simulink model "yaw_damper"  (R2022b)
settings: Solver=VariableStepAuto  StartTime=0.0  StopTime=100  RelTol=1e-3
values from neighbouring files (symbols this model uses):
  G_b_drda = [G_a*G_bdr*(1-k_dr*G_s*G_f*G_rdr_hat), G_a*G_bda-k_dr*G_f*G_s*G_a*G_bdr*G_rda_hat]    [dynamic_SAS_lat.m]
  G_b_drdano = [G_a*G_bdr*(1-k_dr*G_s*G_f*G_rdr_hatno), G_a*G_bda-k_dr*G_f*G_s*G_a*G_bdr*G_rda_hatno]    [dynamic_SAS_lat.m]
  G_phi_drda = [G_a*G_phidr*(1-k_dr*G_s*G_f*G_rdr_hat), G_a*G_phida-k_dr*G_s*G_f*G_a*G_phidr*G_rda_hat]    [dynamic_SAS_lat.m]
  G_phi_drdano = [G_a*G_phidr*(1-k_dr*G_s*G_f*G_rdr_hatno), G_a*G_phida-k_dr*G_s*G_f*G_a*G_phidr*G_rda_hatno]    [dynamic_SAS_lat.m]
libraries: cstblocks x6, simulink_extras x4
settings Model: Creator=mluser  LastModifiedBy=mluser

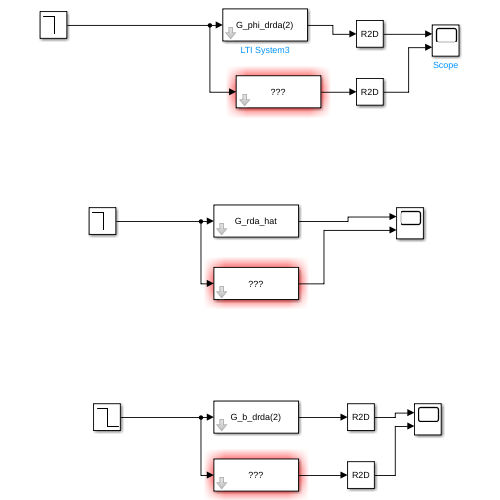
[thumbnail: Simulink's stored preview of the top-level diagram]
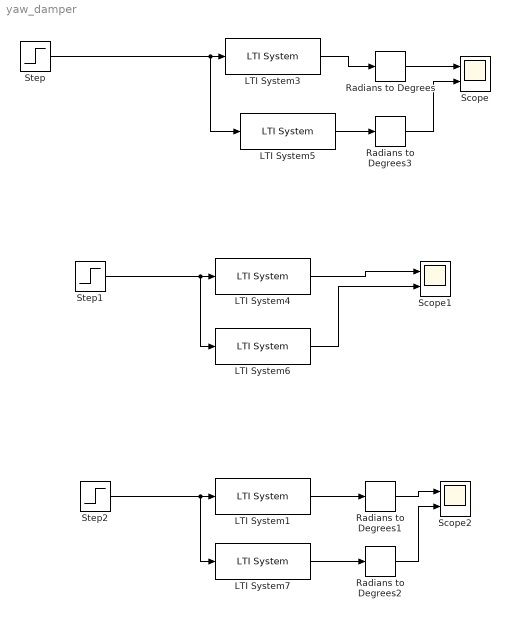
== system yaw_damper ==
  LTI System1 : cstblocks/LTI System  sys=G_b_drda(2)  IC=[]
  LTI System3 : cstblocks/LTI System  sys=G_phi_drda(2)  IC=[]
  LTI System4 : cstblocks/LTI System  sys=G_rda_hat  IC=[]
  LTI System5 : cstblocks/LTI System  sys=G_phi_drdano(2)  IC=[]
  LTI System6 : cstblocks/LTI System  sys=G_rda_hatno  IC=[]
  LTI System7 : cstblocks/LTI System  sys=G_b_drdano(2)  IC=[]
  Radians to Degrees{,1..3} (4 alike) : simulink_extras/Transformations/Radians to Degrees
  Scope : Scope  NumInputPorts=2
  Scope1 : Scope  NumInputPorts=2
  Scope2 : Scope  NumInputPorts=2
  Step : Step  Time=2  Before=1  After=0  SampleTime=0
  Step1 : Step  Time=2  Before=1  After=0  SampleTime=0
  Step2 : Step  Time=2  Before=1  After=0  SampleTime=0
  wires:
  LTI System3/1 -> Radians to Degrees/1
  Step/1 -> LTI System5/1, LTI System3/1
  LTI System4/1 -> Scope1/1
  Step1/1 -> LTI System6/1, LTI System4/1
  LTI System1/1 -> Radians to Degrees1/1
  Step2/1 -> LTI System7/1, LTI System1/1
  Radians to Degrees/1 -> Scope/1
  Radians to Degrees1/1 -> Scope2/1
  LTI System5/1 -> Radians to Degrees3/1
  Radians to Degrees3/1 -> Scope/2
  LTI System6/1 -> Scope1/2
  LTI System7/1 -> Radians to Degrees2/1
  Radians to Degrees2/1 -> Scope2/2
